simulink model "demo5"  (Simulink 3.00)
settings: Solver=ode45  StartTime=0.0  StopTime=10.0  RelTol=1e-3
libraries: roblocks x6, simulink3 x1
settings Model: Creator=pic  LastModifiedBy=pic

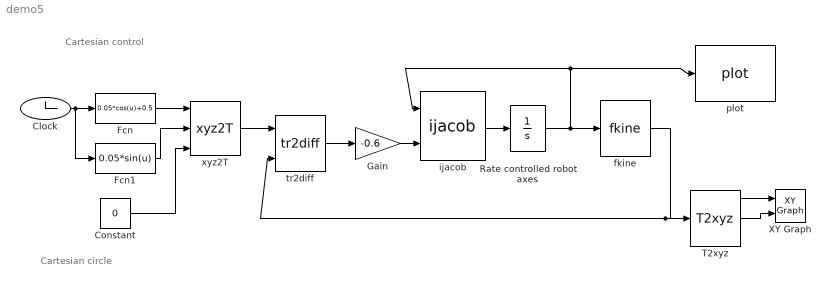
== system demo5 ==
  note: Cartesian circle
  note: Cartesian control
  Clock : Clock
      settings: Decimation=10
  Constant : Constant  Value=0
  Fcn : Fcn  Expr=0.05*cos(u)+0.5
  Fcn1 : Fcn  Expr=0.05*sin(u)
  Gain : Gain  Gain=-0.6  SaturateOnIntegerOverflow=on
  Rate controlled robot axes : Integrator  ExternalReset=none  InitialConditionSource=internal  InitialCondition="[0.2763    0.9125    2.9359         0    2.4348   -0.2763]"  LimitOutput=off  UpperSaturationLimit=inf  LowerSaturationLimit=-inf  ShowSaturationPort=off  ShowStatePort=off  AbsoluteTolerance=auto
  T2xyz : roblocks/T2xyz
  XY Graph : simulink3/Sinks/XY Graph  xmin=-1  xmax=1  ymin=-1  ymax=1  st=-1
  fkine : roblocks/fkine  robot=p560
  ijacob : roblocks/ijacob  robot=p560
  plot : roblocks/plot  robot=p560
  tr2diff : roblocks/tr2diff  robot=robot
  xyz2T : roblocks/xyz2T
  wires:
  Clock/1 -> Fcn/1, Fcn1/1
  Rate controlled robot axes/1 -> fkine/1, ijacob/1, plot/1
  Gain/1 -> ijacob/2
  Constant/1 -> xyz2T/3
  T2xyz/1 -> XY Graph/1
  T2xyz/2 -> XY Graph/2
  tr2diff/1 -> Gain/1
  xyz2T/1 -> tr2diff/1
  fkine/1 -> T2xyz/1, tr2diff/2
  Fcn1/1 -> xyz2T/2
  Fcn/1 -> xyz2T/1
  ijacob/1 -> Rate controlled robot axes/1
